simulink model "parte2_eje3_genclasico"  (R2017b)
settings: Solver=VariableStepAuto  StartTime=0.0  StopTime=10.0  RelTol=1e-3
values from neighbouring files (symbols this model uses):
  H = 3.5    [parte2_ej2_GeneradorBusInfinito.m]    (also in parte2_ej2_GeneradorBusInfinitoHP.m; parte2_eje2_HPModel.m)
  KD = 10    [parte2_ej2_GeneradorBusInfinito.m]    (also in parte2_ej2_GeneradorBusInfinitoHP.m)
  KS = 0.757    [parte2_ej2_GeneradorBusInfinito.m]
settings Model: Creator=Admon  LastModifiedBy=Admon

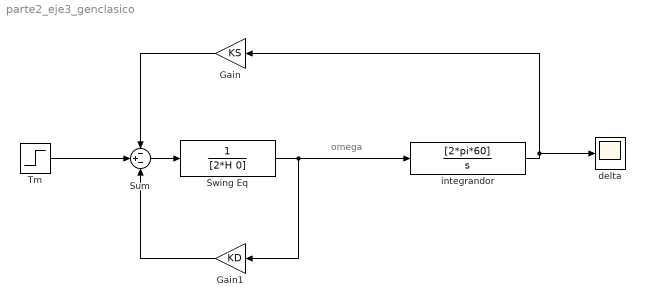
== system parte2_eje3_genclasico ==
  note: omega
  Gain : Gain  Gain=KS
  Gain1 : Gain  Gain=KD
  Sum : Sum  Inputs=-+-
  Swing Eq : TransferFcn  Denominator=[2*H 0]
  Tm : Step  SampleTime=0
  delta : Scope
  integrandor : TransferFcn  Numerator=[2*pi*60]  Denominator=[1 0]
  wires:
  Tm/1 -> Sum/2
  Sum/1 -> Swing Eq/1
  Swing Eq/1 -> Gain1/1, integrandor/1
  Gain1/1 -> Sum/3
  integrandor/1 -> delta/1, Gain/1
  Gain/1 -> Sum/1
